simulink model "NodalAnalysisExample"  (R2024a)
settings: Solver=VariableStepAuto  StartTime=0.0  StopTime=inf  RelTol=1e-6
libraries: fl_lib x16, simulink x11, nesl_utility x7, ee_lib x2
settings Model: Creator=Rocksmithed  LastModifiedBy=callie
settings DebuggingCC: UnconnectedInputMsg=warning  UnconnectedOutputMsg=warning  UnconnectedLineMsg=warning
settings ModelReferenceCC: EnableRefExpFcnMdlSchedulingChecks=on
settings RTWCC: GPUComputeCapability=3.5  DLArmComputeVersion=19.05

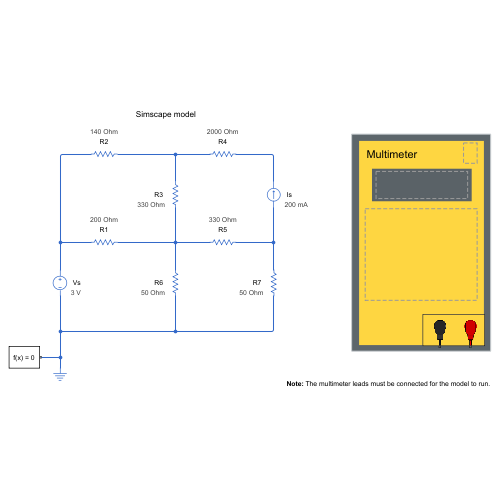
[thumbnail: Simulink's stored preview of the top-level diagram]
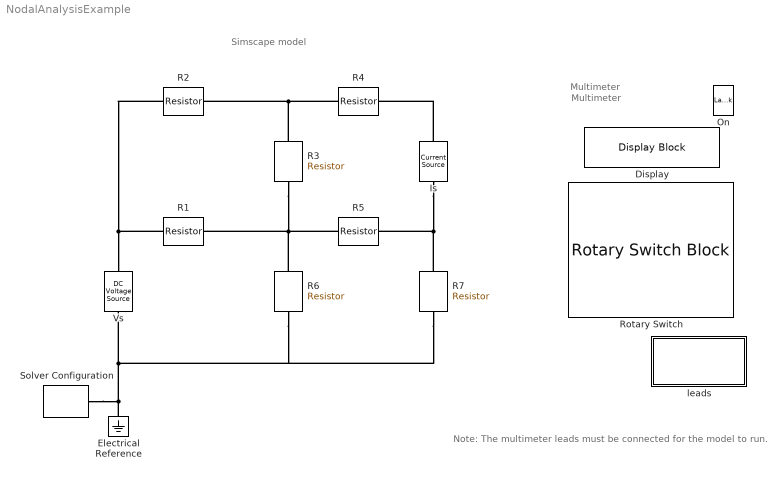
== system NodalAnalysisExample ==
  note: Note: The multimeter leads must be connected for the model to run.
  note: Simscape model
  note: Multimeter
  note: Multimeter
  Display : DisplayBlock  LabelPosition=Hide  Format=Custom  Transparency=1  FormatString=%05.2f
  Electrical Reference : fl_lib/Electrical/Electrical Elements/Electrical Reference
  Is : ee_lib/Sources/Current Source  dc_current=200 mA  ac_current=0 A  ac_shift=0 rad  ac_frequency=60 Hz  noise_mode=0  PSD=0 A^2/Hz  sample_time=1e-3 s  repeatability=1  user_seed=0  auto_seed=1516804514  i_specify=off  i_priority=None  i=0 A  i_nominal_specify=off  i_nominal_value=1  i_nominal_unit=A  v_specify=off  v_priority=None  v=0 V  v_nominal_specify=off  v_nominal_value=1  v_nominal_unit=V
      settings: AttributesFormatString=%<dc_current> %<dc_current_unit>
  On : LampBlock  LabelPosition=Hide
  R1 : fl_lib/Electrical/Electrical Elements/Resistor  R=200 Ohm  i_specify=off  i_priority=None  i=0 A  i_nominal_specify=off  i_nominal_value=1  i_nominal_unit=A  v_specify=off  v_priority=None  v=0 V  v_nominal_specify=off  v_nominal_value=1  v_nominal_unit=V
      settings: AttributesFormatString=%<R> %<R_unit>
  R2 : fl_lib/Electrical/Electrical Elements/Resistor  R=140 Ohm  i_specify=off  i_priority=None  i=0 A  i_nominal_specify=off  i_nominal_value=1  i_nominal_unit=A  v_specify=off  v_priority=None  v=0 V  v_nominal_specify=off  v_nominal_value=1  v_nominal_unit=V
      settings: AttributesFormatString=%<R> %<R_unit>
  R3 : fl_lib/Electrical/Electrical Elements/Resistor  R=330 Ohm  i_specify=off  i_priority=None  i=0 A  i_nominal_specify=off  i_nominal_value=1  i_nominal_unit=A  v_specify=off  v_priority=None  v=0 V  v_nominal_specify=off  v_nominal_value=1  v_nominal_unit=V
      settings: AttributesFormatString=%<R> %<R_unit>
  R4 : fl_lib/Electrical/Electrical Elements/Resistor  R=2000 Ohm  i_specify=off  i_priority=None  i=0 A  i_nominal_specify=off  i_nominal_value=1  i_nominal_unit=A  v_specify=off  v_priority=None  v=0 V  v_nominal_specify=off  v_nominal_value=1  v_nominal_unit=V
      settings: AttributesFormatString=%<R> %<R_unit>
  R5 : fl_lib/Electrical/Electrical Elements/Resistor  R=330 Ohm  i_specify=off  i_priority=None  i=0 A  i_nominal_specify=off  i_nominal_value=1  i_nominal_unit=A  v_specify=off  v_priority=None  v=0 V  v_nominal_specify=off  v_nominal_value=1  v_nominal_unit=V
      settings: AttributesFormatString=%<R> %<R_unit>
  R6 : fl_lib/Electrical/Electrical Elements/Resistor  R=50 Ohm  i_specify=off  i_priority=None  i=0 A  i_nominal_specify=off  i_nominal_value=1  i_nominal_unit=A  v_specify=off  v_priority=None  v=0 V  v_nominal_specify=off  v_nominal_value=1  v_nominal_unit=V
      settings: AttributesFormatString=%<R> %<R_unit>
  R7 : fl_lib/Electrical/Electrical Elements/Resistor  R=50 Ohm  i_specify=off  i_priority=None  i=0 A  i_nominal_specify=off  i_nominal_value=1  i_nominal_unit=A  v_specify=off  v_priority=None  v=0 V  v_nominal_specify=off  v_nominal_value=1  v_nominal_unit=V
      settings: AttributesFormatString=%<R> %<R_unit>
  Rotary Switch : RotarySwitchBlock  LabelPosition=Hide
      settings: Values={{'Off', 'V~', 'V⎓', 'mV⎓', 'Ω', 'A~', 'A⎓', 'mA⎓'}, [0 1 2 3 4 5 6 7]}
  Solver Configuration : nesl_utility/Solver Configuration  PhysicalDomain=network_engine_domain  SubClassName=solver  LeftPortType=input  RightPortType=generic  Tones=[]  Harmonics=[]  SimulateNoise=off  Profile=off  UseLocalSampling=off  EnableSwitchedLinearOptims=on  FrequencyDomain=off  UseCCode=off  RelTol=0.001  AbsTol=1e-06  MinStep=1e-09  ToWorkspace=off  RevertToSquareIcSolve=off  NumHomotopyIterations=100  PhasorMode=off  PhasorModeNumHarmonics=1  ConsistencySolver=NEWTON_FTOL  IndexReductionMethod=DerivativeReplacement  DoDC=off  ResidualTolerance=1e-09  ConsistencyTolSource=GLOBAL  ConsistencyAbsTol=0.001  ConsistencyRelTol=0.001  ConsistencyTolFactor=0.001  UseLocalSolver=off  LocalSolverChoice=NE_BACKWARD_EULER_ADVANCER  ResolveIndetEquations=on  FunctionEvalNumThread=1  LocalSolverSampleTime=0.001  DoFixedCost=off  MaxNonlinIter=3  MaxModeIter=2  ComputeImpulses=off  ImpulseIterations=2  LinearAlgebra=auto  LinearAlgebraNumThread=0  EquationFormulation=NE_TIME_EF  DelaysMemoryBudget=1024  AutomaticFiltering=on  FilteringTimeConstant=0.001  PartitionStorageMethod=AS_NEEDED  PartitionMemoryBudget=1024  PartitionMethod=ROBUST  MultibodyUseLocalSolver=off  MultibodyLocalSolverChoice=ODE1  MultibodyLocalSolverSampleTime=0.001
  Vs : fl_lib/Electrical/Electrical Sources/DC Voltage Source  v0=3 V
      settings: AttributesFormatString=%<v0> %<v0_unit>
  leads : Subsystem  mask(Virtual Multimeter){noise=0}
      mask prompts: noise "Additive noise"
      mask help:
      | Connect the terminals of the multimeter to a Simscape circuit. While the model is running, use the dial to set the measurement type.
      |
      | Note that the model should be running in paced mode.
      settings: PortSchema="{\"entries\":[{\"content\":{\"sides\":[{\"content\":{\"connectorIds\":[]},\"type\":\"ConnectorPlacement.EquallySpacedRectSide\",\"uuid\":\"e6ae0c61-2eb5-460e-b2a2-38a9147b4757\"},{\"content\":{\"connectorIds\":[],\"side\":\"RIGHT\"},\"type\":\"ConnectorPlacement.EquallySpacedRectSide\",\"uuid\":\"ce3a3055-ccd0-4b2b-b818-955585f278b2\"},{\"content\":{\"connectorIds\":[],\"side\":\"TOP\"},\"type\":\"ConnectorPlacement.EquallySpacedRectSide\",\"uuid\":\"55693832-da2d-47ee-8c0b-c43271958a5d\"},{\"content\":{\"connectorIds\":[\"RConn1\",\"RConn2\"],\"side\":\"BOTTOM\"},\"type\":\"ConnectorPlacement.EquallySpacedRectSide\",\"uuid\":\"6e1fba19-6c00-4aec-b19d-3a06ce7f1244\"}]},\"type\":\"ConnectorPlacement.EquallySpacedConnector\",\"uuid\":\"91498f30-f262-43a8-9075-3f461cadc22e\"}],\"packageUris\":[\"http://schema.mathworks.com/mf0/Connector/R2020b\"],\"version\":\"1.0\"}"
      mask Display: image('multimeterLeads.png');
  connections:
  R1/LConn1 -- R2/LConn1 -- Vs/LConn1
  Electrical Reference/LConn1 -- Solver Configuration/RConn1 -- R7/RConn1 -- R6/RConn1 -- Vs/RConn1
  R3/LConn1 -- R4/LConn1 -- R2/RConn1
  R3/RConn1 -- R5/LConn1 -- R6/LConn1 -- R1/RConn1
  R7/LConn1 -- Is/RConn1 -- R5/RConn1
  Is/LConn1 -- R4/RConn1

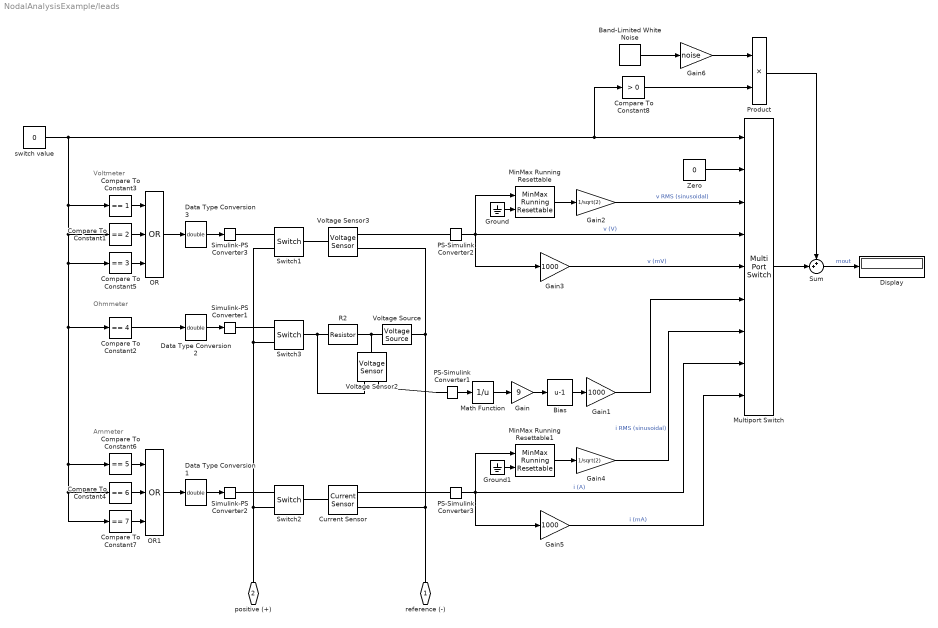
== system NodalAnalysisExample/leads ==
  note: Ohmmeter
  note: Voltmeter
  note: Ammeter
  Band-Limited White Noise : simulink/Sources/Band-Limited White Noise  Cov=1e-2  Ts=0.2  seed=[23341]
  Bias : Bias  Bias=-1  SaturateOnIntegerOverflow=off
  Compare To Constant1 : simulink/Logic and Bit Operations/Compare To Constant  relop===  const=2  OutDataTypeStr=boolean
  Compare To Constant2 : simulink/Logic and Bit Operations/Compare To Constant  relop===  const=4  OutDataTypeStr=boolean
  Compare To Constant3 : simulink/Logic and Bit Operations/Compare To Constant  relop===  const=1  OutDataTypeStr=boolean
  Compare To Constant4 : simulink/Logic and Bit Operations/Compare To Constant  relop===  const=6  OutDataTypeStr=boolean
  Compare To Constant5 : simulink/Logic and Bit Operations/Compare To Constant  relop===  const=3  OutDataTypeStr=boolean
  Compare To Constant6 : simulink/Logic and Bit Operations/Compare To Constant  relop===  const=5  OutDataTypeStr=boolean
  Compare To Constant7 : simulink/Logic and Bit Operations/Compare To Constant  relop===  const=7  OutDataTypeStr=boolean
  Compare To Constant8 : simulink/Logic and Bit Operations/Compare To Constant  relop=>  const=0  OutDataTypeStr=boolean
  Current Sensor : fl_lib/Electrical/Electrical Sensors/Current Sensor
  Data Type Conversion1 : DataTypeConversion  OutDataTypeStr=double  SaturateOnIntegerOverflow=off  RndMeth=Floor
  Data Type Conversion2 : DataTypeConversion  OutDataTypeStr=double  SaturateOnIntegerOverflow=off  RndMeth=Floor
  Data Type Conversion3 : DataTypeConversion  OutDataTypeStr=double  SaturateOnIntegerOverflow=off  RndMeth=Floor
  Display : Display
  Gain : Gain  Gain=9
  Gain1 : Gain  Gain=1000
  Gain2 : Gain  Gain=1/sqrt(2)
  Gain3 : Gain  Gain=1000
  Gain4 : Gain  Gain=1/sqrt(2)
  Gain5 : Gain  Gain=1000
  Gain6 : Gain  Gain=noise
  Ground : Ground
  Ground1 : Ground
  Math Function : Math  Operator=reciprocal
  MinMax Running Resettable : simulink/Math Operations/MinMax Running Resettable  Function=max  vinit=0.0
  MinMax Running Resettable1 : simulink/Math Operations/MinMax Running Resettable  Function=max  vinit=0.0
  Multiport Switch : MultiPortSwitch  DataPortOrder=Zero-based contiguous  Inputs=8  DiagnosticForDefault=None  zeroidx=on  SaturateOnIntegerOverflow=off  InputSameDT=off
  OR : Logic  Operator=OR  Inputs=3  AllPortsSameDT=off  OutDataTypeStr=boolean
  OR1 : Logic  Operator=OR  Inputs=3  AllPortsSameDT=off  OutDataTypeStr=boolean
  PS-Simulink Converter1 : nesl_utility/PS-Simulink Converter  PhysicalDomain=network_engine_domain  SubClassName=ps_output  LeftPortType=input  RightPortType=output  PseudoPeriodic=off  Frequencies=[]  VectorFormat=1-D array  Unit=inherit  AffineConversion=off
  PS-Simulink Converter2 : nesl_utility/PS-Simulink Converter  PhysicalDomain=network_engine_domain  SubClassName=ps_output  LeftPortType=input  RightPortType=output  PseudoPeriodic=off  Frequencies=[]  VectorFormat=1-D array  Unit=inherit  AffineConversion=off
  PS-Simulink Converter3 : nesl_utility/PS-Simulink Converter  PhysicalDomain=network_engine_domain  SubClassName=ps_output  LeftPortType=input  RightPortType=output  PseudoPeriodic=off  Frequencies=[]  VectorFormat=1-D array  Unit=inherit  AffineConversion=off
  Product : Product
  R2 : fl_lib/Electrical/Electrical Elements/Resistor  R=1000 Ohm  i_specify=off  i_priority=None  i=0 A  i_nominal_specify=off  i_nominal_value=1  i_nominal_unit=A  v_specify=off  v_priority=None  v=0 V  v_nominal_specify=off  v_nominal_value=1  v_nominal_unit=V
      settings: AttributesFormatString=%<R> %<R_unit>
  Simulink-PS Converter1 : nesl_utility/Simulink-PS Converter  PhysicalDomain=network_engine_domain  SubClassName=ps_input  LeftPortType=input  RightPortType=output  PseudoPeriodic=off  Frequencies=[]  NoiseDistribution=none  NoiseParameters=[]  Unit=1  AffineConversion=off  FilteringAndDerivatives=provide  SimscapeFilterOrder=1  InputFilterTimeConstant=0.001  UdotUserProvided=0
  Simulink-PS Converter2 : nesl_utility/Simulink-PS Converter  PhysicalDomain=network_engine_domain  SubClassName=ps_input  LeftPortType=input  RightPortType=output  PseudoPeriodic=off  Frequencies=[]  NoiseDistribution=none  NoiseParameters=[]  Unit=1  AffineConversion=off  FilteringAndDerivatives=provide  SimscapeFilterOrder=1  InputFilterTimeConstant=0.001  UdotUserProvided=0
  Simulink-PS Converter3 : nesl_utility/Simulink-PS Converter  PhysicalDomain=network_engine_domain  SubClassName=ps_input  LeftPortType=input  RightPortType=output  PseudoPeriodic=off  Frequencies=[]  NoiseDistribution=none  NoiseParameters=[]  Unit=1  AffineConversion=off  FilteringAndDerivatives=provide  SimscapeFilterOrder=1  InputFilterTimeConstant=0.001  UdotUserProvided=0
  Sum : Sum  Inputs=++|
  Switch1 : fl_lib/Electrical/Electrical Elements/Switch  R_closed=0.01 Ohm  G_open=1e-8 1/Ohm  Threshold=0.5  i_specify=off  i_priority=None  i=0 A  i_nominal_specify=off  i_nominal_value=1  i_nominal_unit=A  v_specify=off  v_priority=None  v=0 V  v_nominal_specify=off  v_nominal_value=1  v_nominal_unit=V
  Switch2 : fl_lib/Electrical/Electrical Elements/Switch  R_closed=0.01 Ohm  G_open=1e-8 1/Ohm  Threshold=0.5  i_specify=off  i_priority=None  i=0 A  i_nominal_specify=off  i_nominal_value=1  i_nominal_unit=A  v_specify=off  v_priority=None  v=0 V  v_nominal_specify=off  v_nominal_value=1  v_nominal_unit=V
  Switch3 : fl_lib/Electrical/Electrical Elements/Switch  R_closed=0.01 Ohm  G_open=1e-8 1/Ohm  Threshold=0.5  i_specify=off  i_priority=None  i=0 A  i_nominal_specify=off  i_nominal_value=1  i_nominal_unit=A  v_specify=off  v_priority=None  v=0 V  v_nominal_specify=off  v_nominal_value=1  v_nominal_unit=V
  Voltage Sensor2 : fl_lib/Electrical/Electrical Sensors/Voltage Sensor
  Voltage Sensor3 : fl_lib/Electrical/Electrical Sensors/Voltage Sensor
  Voltage Source : ee_lib/Sources/Voltage Source  dc_voltage=9 V  ac_voltage=0 V  ac_shift=0 rad  ac_frequency=60 Hz  noise_mode=0  PSD=0 V^2/Hz  sample_time=1e-3 s  repeatability=1  user_seed=0  auto_seed=418932850  i_specify=off  i_priority=None  i=0 A  i_nominal_specify=off  i_nominal_value=1  i_nominal_unit=A  v_specify=off  v_priority=None  v=0 V  v_nominal_specify=off  v_nominal_value=1  v_nominal_unit=V
  Zero : Constant  Value=0
  switch value : Constant  Value=0
  reference (-) : PMIOPort  Side=Right
  positive (+) : PMIOPort  Port=2  Side=Right
  wires:
  Zero/1 -> Multiport Switch/2
  PS-Simulink Converter2/1 -> MinMax Running Resettable/1, Gain3/1, Multiport Switch/4  "v (V)"
  Data Type Conversion2/1 -> Simulink-PS Converter1/1
  Compare To Constant2/1 -> Data Type Conversion2/1
  PS-Simulink Converter1/1 -> Math Function/1
  Bias/1 -> Gain1/1
  Math Function/1 -> Gain/1
  Gain/1 -> Bias/1
  Data Type Conversion3/1 -> Simulink-PS Converter3/1
  Gain2/1 -> Multiport Switch/3  "v RMS (sinusoidal)"
  MinMax Running Resettable/1 -> Gain2/1
  Ground/1 -> MinMax Running Resettable/2
  Compare To Constant3/1 -> OR/1
  Compare To Constant1/1 -> OR/2
  Compare To Constant5/1 -> OR/3
  OR/1 -> Data Type Conversion3/1
  Gain3/1 -> Multiport Switch/5  "v (mV)"
  Gain1/1 -> Multiport Switch/6
  Compare To Constant4/1 -> OR1/2
  MinMax Running Resettable1/1 -> Gain4/1
  Data Type Conversion1/1 -> Simulink-PS Converter2/1
  PS-Simulink Converter3/1 -> Multiport Switch/8, MinMax Running Resettable1/1, Gain5/1  "i (A)"
  switch value/1 -> Compare To Constant8/1, Multiport Switch/1, Compare To Constant7/1, Compare To Constant4/1, Compare To Constant6/1, Compare To Constant2/1, Compare To Constant5/1, Compare To Constant1/1, Compare To Constant3/1
  Ground1/1 -> MinMax Running Resettable1/2
  Compare To Constant7/1 -> OR1/3
  Gain5/1 -> Multiport Switch/9  "i (mA)"
  Gain4/1 -> Multiport Switch/7  "i RMS (sinusoidal)"
  OR1/1 -> Data Type Conversion1/1
  Compare To Constant6/1 -> OR1/1
  Multiport Switch/1 -> Sum/2
  Sum/1 -> Display/1  "mout"
  Product/1 -> Sum/1
  Compare To Constant8/1 -> Product/2
  Band-Limited White Noise/1 -> Gain6/1
  Gain6/1 -> Product/1
  connections:
  R2/RConn1 -- Voltage Sensor2/RConn2 -- Switch3/LConn1
  Switch3/RConn1 -- Simulink-PS Converter1/RConn1
  PS-Simulink Converter1/LConn1 -- Voltage Sensor2/RConn1
  R2/LConn1 -- Voltage Sensor2/LConn1 -- Voltage Source/LConn1
  Switch1/RConn1 -- Simulink-PS Converter3/RConn1
  Voltage Sensor3/LConn1 -- Switch1/LConn1
  PS-Simulink Converter2/LConn1 -- Voltage Sensor3/RConn1
  Current Sensor/LConn1 -- Switch2/LConn1
  Switch1/RConn2 -- Switch3/RConn2 -- Switch2/RConn2 -- positive (+)/RConn1
  Current Sensor/RConn1 -- PS-Simulink Converter3/LConn1
  Voltage Source/RConn1 -- Voltage Sensor3/RConn2 -- Current Sensor/RConn2 -- reference (-)/RConn1
  Switch2/RConn1 -- Simulink-PS Converter2/RConn1
